simulink model "sensorFusionWithControl"  (R2024a)
settings: Solver=FixedStepAuto  StartTime=0.0  StopTime=inf  FixedStep=motorFBRate  RelTol=1e-3
InitFcn:
  | modelParamsDD = Simulink.data.dictionary.open('modelConfigData.sldd');
  | sectModel = getSection(modelParamsDD,'Design Data');
  | contorlRate = getValue(getEntry(sectModel,'controlRate'));
  | 
  | % Complementary filter
  | fc = 10; %Hz
  | tau = 1/(2*pi*fc);
  | alpha = tau/(tau+contorlRate);
  | 
  | % Control params
  | tiltSetPoint = 1; % degree
  | D_min = 50;
  | 
  | % Tilt angle PID
  | Tw = 1;
  | b = 0.05; % lookup table
  | Kp = 35;
  | Ki = 0.005; % At 400 Hz
  | 
  | % Motor params
  | PPR = 13;
  | gearReductionRatio = 42;
  | ABPhase = 2;
  | 
  | % Motor FB params
  | motorFBRate = 0.0002; % 5 kHz
  | wToVolt = 12/(125*2*pi/60); % 125 RPM rated speed
  | Kp_m = 0.01;
  | Ki_m = 0.8;
  | Tw_m = 1;
undefined symbols (not defined in the file): accelToUnit, angleEstRate, controlRate, gyroToUnit, MaxMotorVoltage
libraries: stm32f4xxblockslib x8, stm32f7xxblockslib x2, stm32blockslib x1
settings Model: DataDictionary=globalData.sldd  VariantConfigurationObject=RobotVariantConfig  STM32="{\"I2CControllerWrite\":[{\"ID\":\"sensorFusionWithControl:100\"},{\"ID\":\"sensorFusionWithControl:109\"},{\"ID\":\"sensorFusionWithControl:63:815\"},{\"ID\":\"sensorFusionWithControl:63:816\"},{\"ID\":\"sensorFusionWithControl:78:815\"},{\"ID\":\"sensorFusionWithControl:78:816\"},{\"ID\":\"sensorFusionWithControl:78:817\"}],\"I2CControllerRead\":[{\"ID\":\"sensorFusionWithControl:111\"},{\"ID\":\"sensorFusionWithControl:108\"},{\"ID\":\"sensorFusionWithControl:107\"},{\"ID\":\"sensorFusionWithControl:106\"},{\"ID\":\"sensorFusionWithControl:105\"},{\"ID\":\"sensorFusionWithControl:104\"},{\"ID\":\"sensorFusionWithControl:103\"},{\"ID\":\"sensorFusionWithControl:102\"},{\"ID\":\"sensorFusionWithControl:114\"},{\"ID\":\"sensorFusionWithControl:115\"},{\"ID\":\"sensorFusionWithControl:116\"},{\"ID\":\"sensorFusionWithControl:110\"},{\"ID\":\"sensorFusionWithControl:112\"},{\"ID\":\"sensorFusionWithControl:113\"},{\"ID\":\"sensorFusionWithControl:63:801\"},{\"ID\":\"sensorFusionWithControl:63:802\"},{\"ID\":\"sensorFusionWithControl:63:803\"},{\"ID\":\"sensorFusionWithControl:63:804\"},{\"ID\":\"sensorFusionWithControl:63:799\"},{\"ID\":\"sensorFusionWithControl:63:800\"},{\"ID\":\"sensorFusionWithControl:63:813\"},{\"ID\":\"sensorFusionWithControl:63:814\"},{\"ID\":\"sensorFusionWithControl:78:799\"},{\"ID\":\"sensorFusionWithControl:78:800\"},{\"ID\":\"sensorFusionWithControl:78:801\"},{\"ID\":\"sensorFusionWithControl:78:802\"},{\"ID\":\"sensorFusionWithControl:78:803\"},{\"ID\":\"sensorFusionWithControl:78:804\"},{\"ID\":\"sensorFusionWithControl:78:812\"},{\"ID\":\"sensorFusionWithControl:78:813\"},{\"ID\":\"sensorFusionWithControl:78:814\"}],\"DigitalPortWrite\":[{\"ID\":\"sensorFusionWithControl:197\"},{\"ID\":\"sensorFusionWithControl:199\"},{\"ID\":\"sensorFusionWithControl:201\"},{\"ID\":\"sensorFusionWithControl:203\"},{\"ID\":\"sensorFusionWithControl:667\"},{\"ID\":\"sensorFusionWithControl:668\"},{\"ID\":\"sensorFusionWithControl:669\"},{\"ID\":\"sensorFusionWithControl:670\"},{\"ID\":\"sensorFusionWithControl:778\"},{\"ID\":\"sensorFusionWithControl:779\"},{\"ID\":\"sensorFusionWithControl:780\"},{\"ID\":\"sensorFusionWithControl:781\"},{\"ID\":\"sensorFusionWithControl:790\"},{\"ID\":\"sensorFusionWithControl:791\"},{\"ID\":\"sensorFusionWithControl:792\"},{\"ID\":\"sensorFusionWithControl:793\"},{\"ID\":\"sensorFusionWithControl:1041\"},{\"ID\":\"sensorFusionWithControl:1042\"},{\"ID\":\"sensorFusionWithControl:1043\"},{\"ID\":\"sensorFusionWithControl:1044\"}],\"PWMOutput\":[{\"ID\":\"sensorFusionWithControl:189\"},{\"ID\":\"sensorFusionWithControl:205\"}],\"EncoderBlock\":{\"ID\":\"sensorFusionWithControl:1124\"}}"  SimulationMode=external  Creator=Peter  LastModifiedBy=Peter
settings OptimizationCC: OptimizeBlockIOStorage=off  BufferReuse=off  ReuseModelBlockBuffer=off  GlobalBufferReuse=off  ExpressionFolding=off  EnableMemcpy=off  PassReuseOutputArgsAs=Individual arguments  LocalBlockOutputs=off  ZeroExternalMemoryAtStartup=off  ZeroInternalMemoryAtStartup=off  MaxStackSize=64  OptimizeDataStoreBuffers=off  BusAssignmentInplaceUpdate=off  OptimizationLevel=level0  OptimizationCustomize=off  EfficientTunableParamExpr=on
settings DebuggingCC: ParameterTunabilityLossMsg=error
settings HardwareCC: ProdBitPerPointer=32  ProdBitPerSizeT=32  ProdBitPerPtrDiffT=32  ProdLargestAtomicInteger=Long  ProdLargestAtomicFloat=Double  ProdWordSize=32  ProdLongLongMode=on  ProdHWDeviceType=ARM Compatible->ARM Cortex-M
settings SFSimCC: MATLABDynamicMemAlloc=off
settings RTWCC: Description=Embedded Coder  SystemTargetFile=ert.tlc  HardwareBoard=STM32F7xx Based (Single precision FPU)  TemplateMakefile=ert_default_tmf  Toolchain=GNU Tools for ARM Embedded Processors
settings CodeAppCC: GenerateComments=off  IgnoreCustomStorageClasses=off  OperatorAnnotations=on  SimulinkDataObjDesc=on  SFDataObjDesc=on  SimulinkBlockComments=off
settings ERTTargetCC: TargetLangStandard=C99 (ISO)  CodeReplacementLibrary=ARM Cortex-M  SupportComplex=off  ExtMode=on  ExtModeTransport=3  ExtModeStaticAlloc=on  ExtModeStaticAllocSize=2048  ExtModeMexFile=ext_xcp  ExtModeMexArgs=1 'COM11' 115200  ExtModeIntrfLevel=Level2 - Open

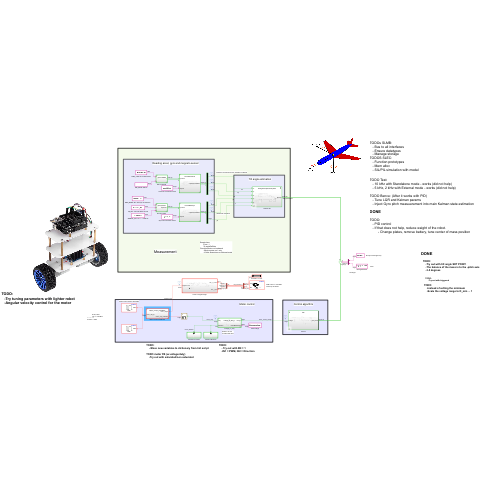
[thumbnail: Simulink's stored preview of the top-level diagram]
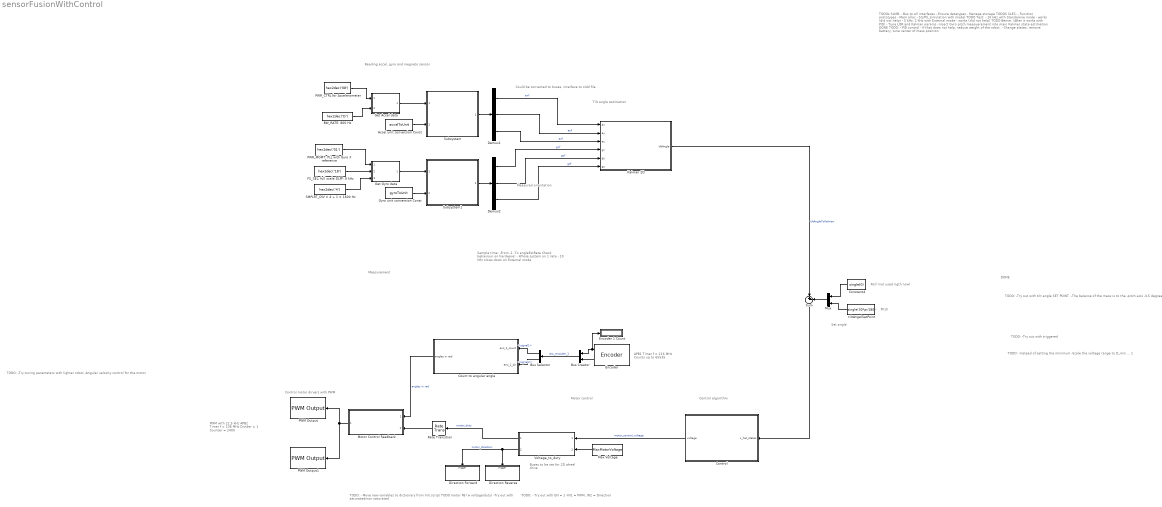
== system sensorFusionWithControl ==
  note: APB1 Timer f = 216 MHz
      | Counts up to 65535
  note: TODO:
      | - Move new variables to dictionary from Init script
      |
      | TODO motor FB (w voltage/duty)
      | -Try out with saturated/non saturated
  note: TODO:
      | -Try tuning parameters with lighter robot
      | -Angular velocity control for the motor
  note: DONE
  note: TODO:
      | -Try out with triggered
  note: Pitch
  note: Roll (not used rigth now)
  note: Set angle
  note: TODO:
      | -Try out with tilt angle SET POINT.
      | -The balance of the mass is to the -pitch axis
      | -3-5 degrees
  note: Measured orientation
  note: TODOs SLMB:
      | - Bus to all interfaces
      | - Ensure datatypes
      | - Manage storage
      | TODOS SLEC:
      | - Function prototypes
      | - Mem alloc
      | - SIL/PIL simulation with model
      |
      | TODO Test:
      | - 10 kHz with Standalone mode - works (did not help)
      | - 5 kHz, 2 kHz with External mode - works (did not help)
      |
      | TODO Bence: (After it works with PID)
      | - Tune LQR and Kalman params
      | - Inject Gyro pitch measuerement into main Kalman state estimation
      |
      | DONE
      |
      | TODO:
      | - PID control
      | - If that does not help, reduce weight of the robot.
      | - Change plates, remove battery, tune center of mass position
  note: PWM with 22,5 kHz
      | APB2 Timer f = 108 MHz
      | Divider = 1
      | Counter = 2400
  note: Sample time:
      | -From -1
      | -To angleEstRate
      | Check behaviour on hardware!
      | - Whole system on 1 rate
      | - 10 kHz slows down on External mode
  note: Measurement
  note: Motor control
  note: Tilt angle estimation
  note: Buses to be set
      | for 2D wheel drive
  note: Control motor dirvers with PWM
  note: Could be converted to buses, interface to sldd file
  note: Reading accel, gyro and megneto sensor
  note: Control algorithm
  note: TODO:
      | -Instead of setting the minimum
      | -Scale the voltage range to D_min ... 1
  note: TODO:
      | - Try out with EN = 1
      | -IN1 = PWM, IN2 = Direction
  Accel unit conversion Const : Constant  Value=accelToUnit  OutDataTypeStr=single
  BW_RATE: 800 Hz : Constant  Value=hex2dec('D')  OutDataTypeStr=uint8
  Bus Creator : BusCreator  Inputs=2
  Bus Selector : BusSelector  OutputSignals=signal1,signal2
  Constant4 : Constant  Value=single(0)
  Control : Subsystem  Variant=on  VariantChoicesEnumeration=controlEnum  VariantControlVariable=controlAlgCtrl  VariantControl=Subsystem2  VariantActivationTime=inherit from Simulink.VariantControl
  Count to angular angle : Subsystem  TreatAsAtomicUnit=on  SystemSampleTime=motorFBRate  VariantControl=encoderDimCtrl == 1
  Demux1 : Demux  Outputs=3
  Demux2 : Demux  Outputs=3
  Direction Forward : Subsystem  TreatAsAtomicUnit=on  SystemSampleTime=controlRate
  Direction Reverse : Subsystem  TreatAsAtomicUnit=on  SystemSampleTime=controlRate
  Encoder : stm32blockslib/Encoder  TimerModule=TIM1  EnableResetInput=off  OutputDirection=on  SampleTime=motorFBRate
      settings: LibrarySourceBlock=stm32f7xxblockslib/Encoder
  Encoder 1 Count : Display
      settings: Format=hex (Stored Integer)
  FS_SEL: full scale DLPF: 8 kHz : Constant  Value=hex2dec('18')  OutDataTypeStr=uint8
  Get Accel data : Subsystem  TreatAsAtomicUnit=on  SystemSampleTime=angleEstRate  ReferencedSubsystem=getAccelData
  Get Gyro data : Subsystem  TreatAsAtomicUnit=on  SystemSampleTime=angleEstRate  ReferencedSubsystem=getGyroData
  Gyro unit conversion Const : Constant  Value=gyroToUnit  OutDataTypeStr=single
  Kalman 2D : Subsystem  Variant=on  VariantChoicesEnumeration=tiltEnum  VariantControlVariable=tiltEstCtrl  VariantControl=Kalman 2D  VariantActivationTime=inherit from Simulink.VariantControl
  Max Voltage : Constant  Value=MaxMotorVoltage  OutDataTypeStr=single
  Motor Control Feedback : Subsystem  TreatAsAtomicUnit=on  SystemSampleTime=motorFBRate  ReferencedSubsystem=Motor_Control_Feedback
  Mux : Mux  Inputs=2
  PWM Output : stm32f7xxblockslib/PWM Output  TimerModule=TIM8  DutycycleUnits=Percentage  EnableChannel1=off  EnableChannel2=off  EnableChannel3=on  EnableChannel4=off  EnableChannel5=off  EnableChannel6=off  EnableCounterInput=off  EnableMainOutputInput=off  EnableFrequencyInput=off  SetRCAfterCE=off  OutputDirection=off  OutputMainOutputEnableStatus=off  SampleTime=0.1  EnableSimPort=off  EnableUpdateEvent=off  EnableCaptureCompare1Event=off  EnableCaptureCompare2Event=off  EnableCaptureCompare3Event=off  EnableCaptureCompare4Event=off  EnableTriggerEvent=off  EnableBreakEvent=off  EnableBreakEvent2=off  ProcessorFamily=STM32F7  hoistedMaskSrc=ECSoC/ECSimCodegen/PWM Output
  PWM Output1 : stm32f7xxblockslib/PWM Output  TimerModule=TIM8  DutycycleUnits=Percentage  EnableChannel1=off  EnableChannel2=off  EnableChannel3=off  EnableChannel4=on  EnableChannel5=off  EnableChannel6=off  EnableCounterInput=off  EnableMainOutputInput=off  EnableFrequencyInput=off  SetRCAfterCE=off  OutputDirection=off  OutputMainOutputEnableStatus=off  SampleTime=0.1  EnableSimPort=off  EnableUpdateEvent=off  EnableCaptureCompare1Event=off  EnableCaptureCompare2Event=off  EnableCaptureCompare3Event=off  EnableCaptureCompare4Event=off  EnableTriggerEvent=off  EnableBreakEvent=off  EnableBreakEvent2=off  ProcessorFamily=STM32F7  hoistedMaskSrc=ECSoC/ECSimCodegen/PWM Output
  PWR_CTRL for Accelerometer : Constant  Value=hex2dec('08')  OutDataTypeStr=uint8
  PWR_MGMT: PLL with Gyro X reference : Constant  Value=hex2dec('01')  OutDataTypeStr=uint8
  Rate Transition : RateTransition  OutPortSampleTime=motorFBRate
  SMPLRT_DIV = 4 + 1 = 1600 Hz : Constant  Value=hex2dec('4')  OutDataTypeStr=uint8
  Subsystem : Subsystem  TreatAsAtomicUnit=on  SystemSampleTime=angleEstRate  ReferencedSubsystem=convertRawAccel
  Subsystem1 : Subsystem  TreatAsAtomicUnit=on  SystemSampleTime=angleEstRate  ReferencedSubsystem=convertRawGyro
  Sum : Sum  Inputs=|+-
  Voltage_to_duty : Subsystem  TreatAsAtomicUnit=on  SystemSampleTime=controlRate  ReferencedSubsystem=Voltage_to_duty_1
  tiltAngelSetPoint : Constant  Value=single(30*pi/180)
  wires:
  Voltage_to_duty/2 -> Direction Reverse/Trigger, Direction Forward/Trigger  "motor_direction"
  Max Voltage/1 -> Voltage_to_duty/2
  Gyro unit conversion Const/1 -> Subsystem1/2
  Subsystem1/1 -> Demux2/1
  PWR_MGMT: PLL with Gyro X reference/1 -> Get Gyro data/1
  Get Gyro data/1 -> Subsystem1/1
  Kalman 2D/1(tiltAngle) -> Sum/1  "tiltAngleToKalman"
  Demux1/1 -> Kalman 2D/1(ax)  "axf"
  Demux1/2 -> Kalman 2D/2(ay)  "ayf"
  Demux1/3 -> Kalman 2D/3(az)  "azf"
  Demux2/3 -> Kalman 2D/6(gz)  "gzf"
  Get Accel data/1 -> Subsystem/1
  Accel unit conversion Const/1 -> Subsystem/2
  Subsystem/1 -> Demux1/1
  Control/1(voltage) -> Voltage_to_duty/1  "motor_control_voltage"
  Demux2/1 -> Kalman 2D/4(gx)  "gxf"
  Demux2/2 -> Kalman 2D/5(gy)  "gyf"
  BW_RATE: 800 Hz/1 -> Get Accel data/2
  PWR_CTRL for Accelerometer/1 -> Get Accel data/1
  FS_SEL: full scale DLPF: 8 kHz/1 -> Get Gyro data/2
  SMPLRT_DIV = 4 + 1 = 1600 Hz/1 -> Get Gyro data/3
  Sum/1 -> Control/1(x_hat_states)
  Mux/1 -> Sum/2
  Constant4/1 -> Mux/1
  tiltAngelSetPoint/1 -> Mux/2
  Encoder/2 -> Bus Creator/2
  Encoder/1 -> Encoder 1 Count/1, Bus Creator/1
  Bus Creator/1 -> Bus Selector/1  "raw_encoder_1"
  Bus Selector/1 -> Count to angular angle/1(enc_1_count)  "<signal1>"
  Bus Selector/2 -> Count to angular angle/2(enc_1_dir)  "<signal2>"
  Motor Control Feedback/1 -> PWM Output1/1, PWM Output/1
  Count to angular angle/1(angles in rad) -> Motor Control Feedback/1  "angles in rad"
  Voltage_to_duty/1 -> Rate Transition/1  "motor_duty"
  Rate Transition/1 -> Motor Control Feedback/2

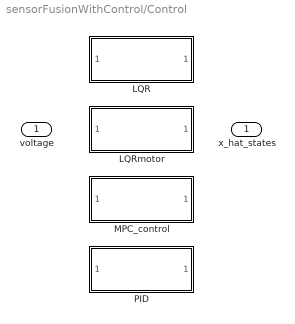
== system sensorFusionWithControl/Control ==
  x_hat_states : Inport  OutDataTypeStr=single
  LQR : Subsystem  TreatAsAtomicUnit=on  SystemSampleTime=controlRate  VariantControl=controlAlgCtrl == controlEnum.LQR  ReferencedSubsystem=LQR
  LQRmotor : Subsystem  TreatAsAtomicUnit=on  SystemSampleTime=controlRate  VariantControl=controlAlgCtrl == controlEnum.LQRmotor  ReferencedSubsystem=LQRmotor
  MPC_control : Subsystem  TreatAsAtomicUnit=on  SystemSampleTime=controlRate  VariantControl=controlAlgCtrl == controlEnum.MPC_control  ReferencedSubsystem=MPC_control
  PID : Subsystem  TreatAsAtomicUnit=on  SystemSampleTime=controlRate  VariantControl=controlAlgCtrl == controlEnum.PID  ReferencedSubsystem=PID
  voltage : Outport  OutDataTypeStr=single

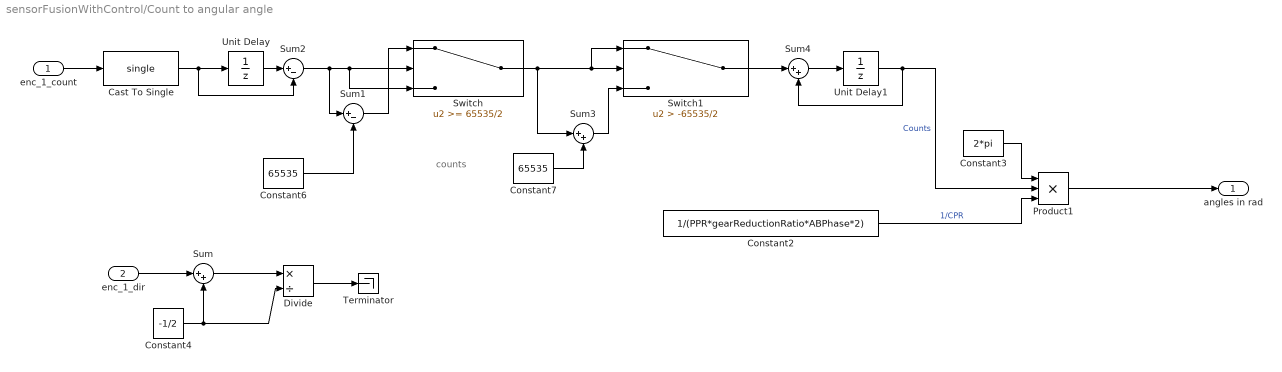
== system sensorFusionWithControl/Count to angular angle ==
  note: counts
  enc_1_count : Inport
  enc_1_dir : Inport  Port=2
  Cast To Single : DataTypeConversion  OutDataTypeStr=single  SaturateOnIntegerOverflow=off  RndMeth=Floor
  Constant2 : Constant  Value=1/(PPR*gearReductionRatio*ABPhase*2)  OutDataTypeStr=single
  Constant3 : Constant  Value=2*pi  OutDataTypeStr=single
  Constant4 : Constant  Value=-1/2  OutDataTypeStr=single
  Constant6 : Constant  Value=65535  OutDataTypeStr=single
  Constant7 : Constant  Value=65535  OutDataTypeStr=single
  Divide : Product  Inputs=*/  OutDataTypeStr=single
  Product1 : Product  Inputs=3  OutDataTypeStr=single
  Sum : Sum  Inputs=|++  OutDataTypeStr=single
  Sum1 : Sum  Inputs=|+-
  Sum2 : Sum  Inputs=|+-  OutDataTypeStr=single  AccumDataTypeStr=single
  Sum3 : Sum  Inputs=|++
  Sum4 : Sum  Inputs=|++
  Switch : Switch  Threshold=65535/2  SaturateOnIntegerOverflow=off  InputSameDT=off
  Switch1 : Switch  Criteria=u2 > Threshold  Threshold=-65535/2  SaturateOnIntegerOverflow=off  InputSameDT=off
  Terminator : Terminator
  Unit Delay : UnitDelay  SampleTime=-1  HasFrameUpgradeWarning=on
  Unit Delay1 : UnitDelay  SampleTime=-1  HasFrameUpgradeWarning=on
  angles in rad : Outport  OutDataTypeStr=single
  wires:
  Constant2/1 -> Product1/3  "1/CPR"
  Constant3/1 -> Product1/1
  enc_1_dir/1 -> Sum/1
  Constant4/1 -> Sum/2, Divide/2
  Sum/1 -> Divide/1
  Product1/1 -> angles in rad/1
  Constant6/1 -> Sum1/2
  Sum1/1 -> Switch/1
  Sum2/1 -> Sum1/1, Switch/3, Switch/2
  Unit Delay/1 -> Sum2/1
  Switch/1 -> Sum3/1, Switch1/1, Switch1/2
  Constant7/1 -> Sum3/2
  Sum3/1 -> Switch1/3
  Switch1/1 -> Sum4/1
  Sum4/1 -> Unit Delay1/1
  Unit Delay1/1 -> Sum4/2, Product1/2  "Counts"
  Cast To Single/1 -> Sum2/2, Unit Delay/1
  enc_1_count/1 -> Cast To Single/1
  Divide/1 -> Terminator/1

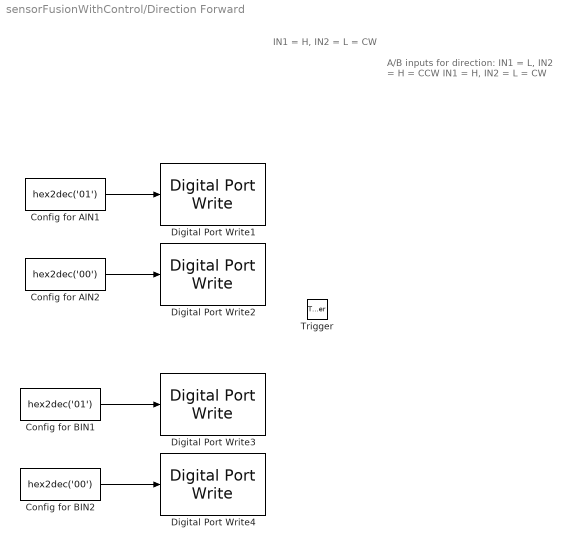
== system sensorFusionWithControl/Direction Forward ==
  note: A/B inputs for direction:
      | IN1 = L, IN2 = H = CCW
      | IN1 = H, IN2 = L = CW
  note: IN1 = H, IN2 = L = CW
  Trigger : TriggerPort  VariantControl=(inherit)  PortDimensions=1
  Config for AIN1 : Constant  Value=hex2dec('01')  OutDataTypeStr=uint8
  Config for AIN2 : Constant  Value=hex2dec('00')  OutDataTypeStr=uint8
  Config for BIN1 : Constant  Value=hex2dec('01')  OutDataTypeStr=uint8
  Config for BIN2 : Constant  Value=hex2dec('00')  OutDataTypeStr=uint8
  Digital Port Write1 : stm32f4xxblockslib/Digital Port Write  PortName=GPIOA  PinNumber=[3]  ReadOperation=off  IOAsArray=off  EnableSimPort=off  hoistedMaskSrc=ECSoC/ECSimCodegen/Digital Port Write
      settings: LibrarySourceBlock=stm32f7xxblockslib/Digital Port Write
  Digital Port Write2 : stm32f4xxblockslib/Digital Port Write  PortName=GPIOC  PinNumber=[0]  ReadOperation=off  IOAsArray=off  EnableSimPort=off  hoistedMaskSrc=ECSoC/ECSimCodegen/Digital Port Write
      settings: LibrarySourceBlock=stm32f7xxblockslib/Digital Port Write
  Digital Port Write3 : stm32f4xxblockslib/Digital Port Write  PortName=GPIOC  PinNumber=[10]  ReadOperation=off  IOAsArray=off  EnableSimPort=off  hoistedMaskSrc=ECSoC/ECSimCodegen/Digital Port Write
      settings: LibrarySourceBlock=stm32f7xxblockslib/Digital Port Write
  Digital Port Write4 : stm32f4xxblockslib/Digital Port Write  PortName=GPIOF  PinNumber=[14]  ReadOperation=off  IOAsArray=off  EnableSimPort=off  hoistedMaskSrc=ECSoC/ECSimCodegen/Digital Port Write
      settings: LibrarySourceBlock=stm32f7xxblockslib/Digital Port Write
  wires:
  Config for BIN2/1 -> Digital Port Write4/1
  Config for AIN2/1 -> Digital Port Write2/1
  Config for BIN1/1 -> Digital Port Write3/1
  Config for AIN1/1 -> Digital Port Write1/1

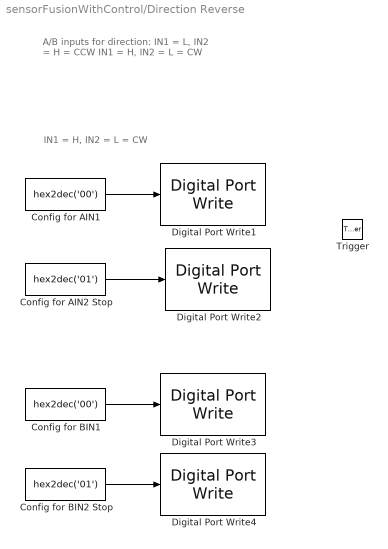
== system sensorFusionWithControl/Direction Reverse ==
  note: A/B inputs for direction:
      | IN1 = L, IN2 = H = CCW
      | IN1 = H, IN2 = L = CW
  note: IN1 = H, IN2 = L = CW
  Trigger : TriggerPort  TriggerType=falling  VariantControl=(inherit)  PortDimensions=1
  Config for AIN1 : Constant  Value=hex2dec('00')  OutDataTypeStr=uint8
  Config for AIN2 Stop : Constant  Value=hex2dec('01')  OutDataTypeStr=uint8
  Config for BIN1 : Constant  Value=hex2dec('00')  OutDataTypeStr=uint8
  Config for BIN2 Stop : Constant  Value=hex2dec('01')  OutDataTypeStr=uint8
  Digital Port Write1 : stm32f4xxblockslib/Digital Port Write  PortName=GPIOA  PinNumber=[3]  ReadOperation=off  IOAsArray=off  EnableSimPort=off  hoistedMaskSrc=ECSoC/ECSimCodegen/Digital Port Write
      settings: LibrarySourceBlock=stm32f7xxblockslib/Digital Port Write
  Digital Port Write2 : stm32f4xxblockslib/Digital Port Write  PortName=GPIOC  PinNumber=[0]  ReadOperation=off  IOAsArray=off  EnableSimPort=off  hoistedMaskSrc=ECSoC/ECSimCodegen/Digital Port Write
      settings: LibrarySourceBlock=stm32f7xxblockslib/Digital Port Write
  Digital Port Write3 : stm32f4xxblockslib/Digital Port Write  PortName=GPIOC  PinNumber=[10]  ReadOperation=off  IOAsArray=off  EnableSimPort=off  hoistedMaskSrc=ECSoC/ECSimCodegen/Digital Port Write
      settings: LibrarySourceBlock=stm32f7xxblockslib/Digital Port Write
  Digital Port Write4 : stm32f4xxblockslib/Digital Port Write  PortName=GPIOF  PinNumber=[14]  ReadOperation=off  IOAsArray=off  EnableSimPort=off  hoistedMaskSrc=ECSoC/ECSimCodegen/Digital Port Write
      settings: LibrarySourceBlock=stm32f7xxblockslib/Digital Port Write
  wires:
  Config for AIN1/1 -> Digital Port Write1/1
  Config for BIN1/1 -> Digital Port Write3/1
  Config for BIN2 Stop/1 -> Digital Port Write4/1
  Config for AIN2 Stop/1 -> Digital Port Write2/1

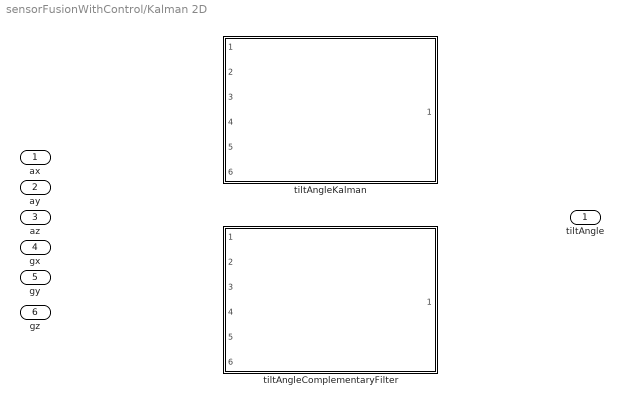
== system sensorFusionWithControl/Kalman 2D ==
  ax : Inport
  ay : Inport  Port=2
  az : Inport  Port=3
  gx : Inport  Port=4
  gy : Inport  Port=5
  gz : Inport  Port=6
  tiltAngleComplementaryFilter : Subsystem  TreatAsAtomicUnit=on  SystemSampleTime=controlRate  VariantControl=tiltEstCtrl == tiltEnum.tiltAngleComplementaryFilter  ReferencedSubsystem=tiltAngleComplementaryFilter
  tiltAngleKalman : Subsystem  TreatAsAtomicUnit=on  SystemSampleTime=angleEstRate  VariantControl=tiltEstCtrl == tiltEnum.tiltAngleKalman  ReferencedSubsystem=tiltAngleKalman
  tiltAngle : Outport
